simulink model "multidim_multimodel_lvl2"  (R2019b)
settings: Solver=FixedStepAuto  StartTime=0.0  StopTime=100  FixedStep=0.005  RelTol=1e-3
model workspace (MAT data in the model file):
  P = [1.1  0.1; 0.1  0.1]
  alpha_hat_init = Simulink.Parameter
  alpha_hat_init.Value = [0.7; 0.1]
  alpha_hat_init.DataType = 'auto'
  alpha_hat_init.Dimensions = [2 1]
  gamma = Simulink.Parameter
  gamma.Value = 1.4
  gamma.DataType = 'auto'
  gamma.Dimensions = [1 1]
  theta_i_init = Simulink.Parameter
  theta_i_init.Value = [-15  15  -10; 10  15  -10]
  theta_i_init.DataType = 'auto'
  theta_i_init.Dimensions = [2 3]
  theta_m = Simulink.Parameter
  theta_m.Value = [-5; -6]
  theta_m.DataType = 'auto'
  theta_m.Dimensions = [2 1]
  theta_p = Simulink.Parameter
  theta_p.Value = [-2; 9]
  theta_p.DataType = 'auto'
  theta_p.Dimensions = [2 1]
settings Model: Creator=luthraj  LastModifiedBy=darkapex

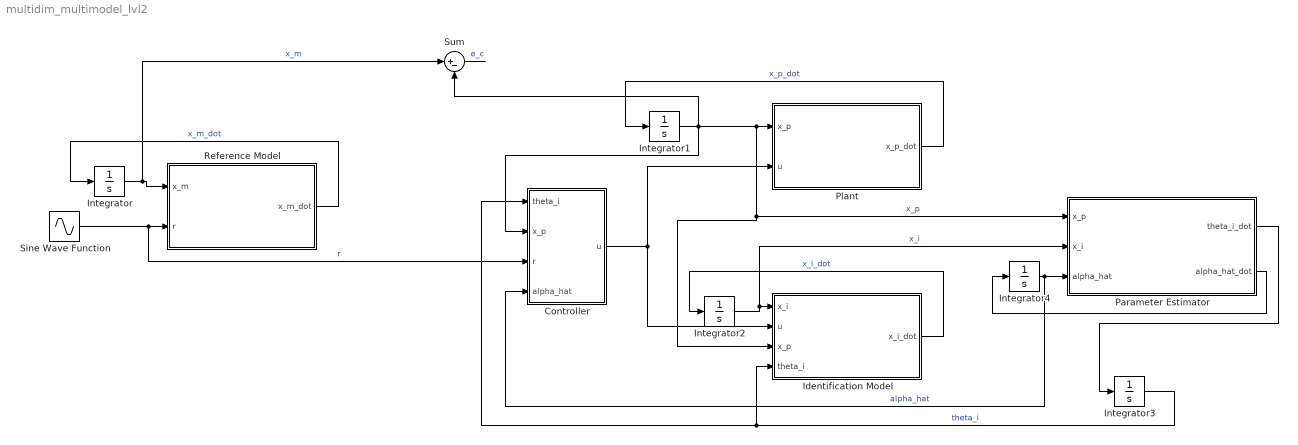
== system multidim_multimodel_lvl2 ==
  Controller : MATLAB Function  TreatAsAtomicUnit=on
  Identification Model : MATLAB Function  TreatAsAtomicUnit=on
  Integrator : Integrator  InitialCondition=zeros(size(theta_m))
  Integrator1 : Integrator  InitialCondition=zeros(size(theta_p))
  Integrator2 : Integrator  InitialCondition=zeros(size(theta_i_init))
  Integrator3 : Integrator  InitialCondition=theta_i_init
  Integrator4 : Integrator  InitialCondition=alpha_hat_init
  Parameter Estimator : MATLAB Function  TreatAsAtomicUnit=on
  Plant : MATLAB Function  TreatAsAtomicUnit=on
  Reference Model : MATLAB Function  TreatAsAtomicUnit=on
  Sine Wave Function : Sin  Amplitude=5  Frequency=0.2*pi  SampleTime=0
  Sum : Sum  Inputs=|+-
  wires:
  Reference Model/1(x_m_dot) -> Integrator/1  "x_m_dot"
  Integrator/1 -> Sum/1, Reference Model/1(x_m)  "x_m"
  Sine Wave Function/1 -> Controller/3(r), Reference Model/2(r)  "r"
  Integrator1/1 -> Sum/2, Controller/2(x_p), Identification Model/3(x_p), Parameter Estimator/1(x_p), Plant/1(x_p)  "x_p"
  Plant/1(x_p_dot) -> Integrator1/1  "x_p_dot"
  Identification Model/1(x_i_dot) -> Integrator2/1  "x_i_dot"
  Integrator2/1 -> Parameter Estimator/2(x_i), Identification Model/1(x_i)  "x_i"
  Parameter Estimator/1(theta_i_dot) -> Integrator3/1
  Integrator3/1 -> Controller/1(theta_i), Identification Model/4(theta_i)  "theta_i"
  Controller/1(u) -> Plant/2(u), Identification Model/2(u)
  Sum/1 -> ?  "e_c"
  Parameter Estimator/2(alpha_hat_dot) -> Integrator4/1
  Integrator4/1 -> Controller/4(alpha_hat), Parameter Estimator/3(alpha_hat)  "alpha_hat"

== matlab function multidim_multimodel_lvl2/Plant ==
  data: x_p input; u input; x_p_dot output; theta_p parameter
function x_p_dot = plant(x_p, u, theta_p)
A_p = companion(theta_p);
b = zeros(size(x_p));
b(end) = 1;
x_p_dot = A_p * x_p + b*u;


function A_m = companion(theta)
theta_ = [1; -rot90(theta, 2)];
A_m = rot90(compan(theta_), 2);

== matlab function multidim_multimodel_lvl2/Reference Model ==
  data: x_m input; r input; x_m_dot output; theta_m parameter
function x_m_dot = reference(x_m, r, theta_m)
A_m = companion(theta_m);
b = zeros(size(x_m));
b(end) = 1;
x_m_dot = A_m * x_m + b*r;


function A_m = companion(theta)
theta_ = [1; -rot90(theta, 2)];
A_m = rot90(compan(theta_), 2);

== matlab function multidim_multimodel_lvl2/Identification Model ==
  data: x_i input; u input; x_p input; x_i_dot output; theta_i input; theta_m parameter
function x_i_dot = ident(x_i, u, x_p, theta_i, theta_m)
n = size(theta_i, 2); % no of models
x_i_dot = zeros(size(x_i));
b = zeros(size(theta_i, 1), 1); % order of model
b(end) = 1;
A_m = companion(theta_m);
for i = 1:n
    A_i = companion(theta_i(:, i));
    x_i_dot(:, i) = A_m * x_i(:, i) + (A_i - A_m) * x_p + b*u;
end

function A_m = companion(theta)
theta_ = [1; -rot90(theta, 2)];
A_m = rot90(compan(theta_), 2);

== matlab function multidim_multimodel_lvl2/Controller ==
  data: u output; theta_i input; x_p input; r input; theta_m parameter; alpha_hat input
function u = controller(theta_i, x_p, r, theta_m, alpha_hat)
alpha = [alpha_hat; 1-sum(alpha_hat)];
theta_0 = theta_i * alpha;
k = theta_0 - theta_m;
u = -k' * x_p + r;

== matlab function multidim_multimodel_lvl2/Parameter Estimator ==
  data: theta_i_dot output; x_p input; x_i input; alpha_hat input; P parameter; gamma parameter; alpha_hat_dot output
function [theta_i_dot, alpha_hat_dot] = estimator(x_p, x_i, alpha_hat, P, gamma)
n = size(x_i, 2); % no of models

% theta estimate
theta_i_dot = zeros(size(x_i));
b = zeros(size(x_p));
b(end) = 1;
for i = 1:n
    e_i = x_i(:,i) - x_p;
    theta_i_dot(:,i) = -gamma * e_i' * P * b * x_p;
end

% alpha estimate
E_hat = zeros(n-1);
h = -(x_i(:, n) - x_p); % h = -e_n
for i = 1:(n-1)
    e_i = x_i(:,i) - x_p;
    E_hat(:, i) = e_i + h;
end
alpha_hat_dot = -E_hat' * E_hat * alpha_hat + E_hat' * h;
